simulink library "mesh_assembly_library"  (R2021a)
settings: Solver=VariableStepAuto  StartTime=0.0  StopTime=10.0  RelTol=1e-3
undefined symbols (not defined in the file): X, Y, Z
libraries: sm_lib x71, $bdroot x8, nesl_utility x6, Contact_Forces_Lib x1
(part 1 of 3)
settings Model: Creator=Daniel Adejumo  LastModifiedBy=Daniel Adejumo

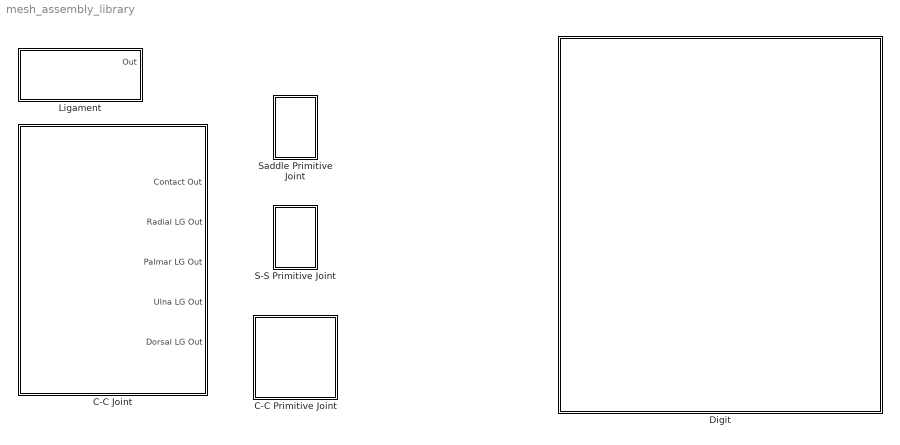
== system mesh_assembly_library ==
  C-C Joint : Subsystem  mask(Cylinder in Cylinder - DARM IP Joint){distal_arc_radius=0, proximal_arc_radius=0, active_range=[-60, 60], initial_rotation=0, distal_ring_thickness=1/1000, distal_surface_length=10/1000, distal_surface_thickness=0.1/1000, proximal_surface_length=10/1000, proximal_surface_thickness=0.1/1000, visual_color=[0.9 0.2 0.2], visual_opacity=0.7, contact_stiffness=1e4, contact_damping=1e2, coefficient_kinetic_friction=0.1, coefficient_static_friction=0.2, velocity_threshold=0.001, lg_tension_stiffness=0, lg_tension_damping_coefficient=0, lg_transition_region_width=1e-3, lg_density=0, lg_damping=0, radial_lg_dim=[0, 0, 0], palmar_lg_dim=[0, 0, 0], ulnar_lg_dim=[0, 0, 0], dorsal_lg_dim=[0, 0, 0]}
      mask prompts: distal_arc_radius "Distal Arc Radius [m]"; proximal_arc_radius "Proximal Arc Radius [m]"; active_range "Active Range (min, max angle) [deg]"; initial_rotation "Initial Rotation [deg]"; distal_ring_thickness "Distal Ring Thickness [m]"; distal_surface_length "Distal Surface Length [m]"; distal_surface_thickness "Distal Surface Thickness [m]"; proximal_surface_length "Proximal Surface Length [m]"; proximal_surface_thickness "Proximal Surface Thickness [m]"; visual_color "Visual Colour [RGB]"; visual_opacity "Visual Opacity (0 - 1)"; contact_stiffness "Contact Stiffness [N/m]"; contact_damping "Contact Damping [N/(m/s)]"; coefficient_kinetic_friction "Coefficient of Kinetic Friction"; coefficient_static_friction "Coefficient of Static Friction"; velocity_threshold "Velocity Threshold [m/s]"; lg_tension_stiffness "Tension Stiffness [N/m]"; lg_tension_damping_coefficient "Tension Damping Coefficient [N/(m/s)]"; lg_transition_region_width "Transition Region Width [m]"; lg_density "Density [Kg/m^3]"; lg_damping "Damping [N/(m/s)]"; radial_lg_dim "Dimensions (L, W, T) [m]"; palmar_lg_dim "Dimensions (L, W, T) [m]"; ulnar_lg_dim "Dimensions (L, W, T) [m]"; dorsal_lg_dim "Dimensions (L, W, T) [m]"
      mask help: The Cylinder in Cylinder Joint models a 1-DOF joint found in the interphalangeal articulation.
      settings: PortSchema="{\"entries\":[{\"content\":{\"sides\":[{\"content\":{\"connectorIds\":[\"LConn1\",\"LConn2\",\"LConn3\",\"LConn4\",\"LConn5\",\"LConn6\",\"LConn7\",\"LConn8\"]},\"type\":\"ConnectorPlacement.EquallySpacedRectSide\",\"uuid\":\"de75d0fa-dcb7-4671-a193-b6d8e2533622\"},{\"content\":{\"connectorIds\":[\"RConn1\",\"Out1\",\"Out2\",\"Out3\",\"Out4\",\"Out5\",\"RConn2\"],\"side\":\"RIGHT\"},\"type\":\"ConnectorPlacement.EquallySpacedRectSide\",\"uuid\":\"61947ab9-5bc1-4fe7-b694-bbba1acc34a0\"},{\"content\":{\"connectorIds\":[],\"side\":\"TOP\"},\"type\":\"ConnectorPlacement.EquallySpacedRectSide\",\"uuid\":\"94257d25-1dd3-43a0-827d-d6eeaffa38d1\"}]},\"type\":\"ConnectorPlacement.EquallySpacedConnector\",\"uuid\":\"ad636cf9-9422-4be4-a938-719e0f4b0058\"}],\"packageUris\":[\"http://schema.mathworks.com/mf0/Connector/R2020b\"],\"version\":\"1.0\"}"
      mask Help:
      | <p>The Cylinder in Cylinder Joint models a 1-DOF joint found in the interphalangeal articulation. </p>
      | 
      | <h3> Port Names: </h3>
      | 
      | <p><i>Radial LG Head_R:</i> Radial aspect of the head of the radial ligament</p>
      | <p><i>Radial LG Head_U:</i> Ulnar aspect of the head of the radial ligament</p>
      mask DialogControl DescGroupVar Prompt: Cylinder in Cyclinder Joint
      mask DialogControl DescTextVar Prompt: The Distal Arc Radius is the radius of its inner circle. The Proximal arc radius is the radius of its outer circle.
      mask DialogControl geometry Prompt: Geometry
      mask DialogControl visual Prompt: Visual
      mask DialogControl contact Prompt: Contact
      mask DialogControl Container13 Prompt: Ligaments
      mask DialogControl Container21 Prompt: Mechanics
      mask DialogControl Container20 Prompt: Geometry
      mask DialogControl Container16 Prompt: Radial Collateral Ligament
      mask DialogControl Container16_copy Prompt: Palmar Ligament
      mask DialogControl Container16_copy_copy Prompt: Ulnar Collateral Ligament
      mask DialogControl Container16_copy_copy_copy Prompt: Dorsal Ligament
  C-C Primitive Joint : Subsystem  mask{stiffness=0, damping=0, lower_limit=-90, upper_limit=90, initial_position=0, radius=0, length=0, thickness=0, color=[1.0 0.0 0.0], opacity=1.0}
      mask prompts: stiffness "Stiffness [Nm/deg]"; damping "Damping [Nm/(deg/s)]"; lower_limit "Lower Limit [deg]"; upper_limit "Upper Limit [deg]"; initial_position "Initial Position [deg]"; radius "Radius [m]"; length "Length [m]"; thickness "Thickness [m]"; color "Color (RGB - Range [0, 1])"; opacity "Opacity (Range [0, 1])"
      mask DialogControl DescGroupVar Prompt: C-C Primitive Joint
      mask DialogControl DescTextVar Prompt: Primitive representation of a cylinder to cylinder joint using a simple revolute joint. This joint is found in at the PIP and DIP joints.
      mask DialogControl Container4 Prompt: Mechanics
      mask DialogControl Container6 Prompt: Visualization
  Digit : Subsystem  mask{links_density=1000, distal_phalanx="", distal_phalanx_base=[[0 0 0]; [0 0 0]], distal_phalanx_dip_joint=[[0 0 0]; [0 0 0]], distal_phalanx_head=[[0 0 0]; [0 0 0]], middle_phalanx="", middle_phalanx_base=[[0 0 0]; [0 0 0]], middle_phalanx_pip_joint=[[0 0 0]; [0 0 0]], middle_phalanx_head=[[0 0 0]; [0 0 0]], middle_phalanx_dip_joint=[[0 0 0]; [0 0 0]], proximal_phalanx="", proximal_phalanx_base=[[0 0 0]; [0 0 0]], proximal_phalanx_mcp_joint=[[0 0 0]; [0 0 0]], proximal_phalanx_head=[[0 0 0]; [0 0 0]], proximal_phalanx_pip_joint=[[0 0 0]; [0 0 0]], metacarpal="", metacarpal_base=[[0 0 0]; [0 0 0]], metacarpal_cm_joint=[[0 0 0]; [0 0 0]], metacarpal_head=[[0 0 0]; [0 0 0]], metacarpal_mcp_joint=[[0 0 0]; [0 0 0]], mcp_viz_radius=0, mcp_viz_color=[1.0 0.0 0.0], mcp_viz_opacity=1.0, pip_viz_radius=0, pip_viz_length=0, pip_viz_thickness=0, pip_viz_color=[1.0 0.0 0.0], pip_viz_opacity=1.0, dip_viz_radius=0, dip_viz_length=0, dip_viz_thickness=0, dip_viz_color=[1.0 0.0 0.0], dip_viz_opacity=1.0}
      mask prompts: links_density "Density [Kg/(m^3)]"; distal_phalanx "File Name"; distal_phalanx_base "Base Transform (Translation [m], Rotation: X-Y-Z [deg])"; distal_phalanx_dip_joint "DIP Joint Transform (Translation, Rotation)"; distal_phalanx_head "Head Transform (Translation, Rotation)"; middle_phalanx "File Name"; middle_phalanx_base "Base Transform"; middle_phalanx_pip_joint "PIP Joint Transform"; middle_phalanx_head "Head Transform"; middle_phalanx_dip_joint "DIP Joint Transform"; proximal_phalanx "File Name"; proximal_phalanx_base "Base Transform"; proximal_phalanx_mcp_joint "MCP Joint Transform"; proximal_phalanx_head "Head Transform"; proximal_phalanx_pip_joint "PIP Joint Transform"; metacarpal "File Name"; metacarpal_base "Base Transform"; metacarpal_cm_joint "CM Joint Transform"; metacarpal_head "Head Transform"; metacarpal_mcp_joint "MCP Joint Transform"; mcp_viz_radius "Radius [m]"; mcp_viz_color "Color (RGB - Range [0, 1])"; mcp_viz_opacity "Opacity (Range [0, 1])"; pip_viz_radius "Radius [m]"; pip_viz_length "Length [m]"; pip_viz_thickness "Thickness [m]"; pip_viz_color "Color (RGB - Range [0, 1])"; pip_viz_opacity "Opacity (Range [0, 1])"; dip_viz_radius "Radius [m]"; dip_viz_length "Length [m]"; dip_viz_thickness "Thickness [m]"; dip_viz_color "Color (RGB - Range [0, 1])"; dip_viz_opacity "Opacity (Range [0, 1])"
      mask DialogControl DescGroupVar Prompt: Digit Subsystem
      mask DialogControl DescTextVar Prompt: This subsystem encapsulates the bones and joints that makes up digits II - V. Metacarpal bone, Proximal, Middle and Distal Phalanxes; MCP, PIP and DIP Joints.
      mask DialogControl Links Prompt: Links
      mask DialogControl Distal_Phalanx Prompt: Distal Phalanx
      mask DialogControl Middle_Phalanx Prompt: Middle Phalanx
      mask DialogControl Proximal_Phalanx Prompt: Proximal Phalanx
      mask DialogControl Metacarpal Prompt: Metacarpal
      mask DialogControl Container10 Prompt: Visualization
      mask DialogControl Container11 Prompt: MCP Joint
      mask DialogControl Container12 Prompt: PIP Joint
      mask DialogControl Container13 Prompt: DIP Joint
  Ligament : Subsystem  Variant=on  mask{length=0.4, width=0.08, thickness=0.008, tension_stiffness=35E3, tension_damping_coefficient=100, transition_region_width=1e-3, density=800, damping_coefficient=0.2}
      mask prompts: length "Length [m]"; width "Width [m]"; thickness "Thickness [m]"; tension_stiffness "Tension Stiffness [N/m]"; tension_damping_coefficient "Tension Damping Coefficient [N/(m/s)]"; transition_region_width "Transition Region Width [m]"; density "Density [Kg/m^3]"; damping_coefficient "Damping [N/(m/s)]"
      mask DialogControl geometry Prompt: Geometry Parameters
      mask DialogControl mechanics Prompt: Mechanics Parameters
  S-S Primitive Joint : Subsystem  mask{stiffness=0, damping=0, x_limits=[-90 90], y_limits=[-90 90], x_initial_position=0, y_initial_position=0, radius=0, color=[1.0 0.0 0.0], opacity=1.0}
      mask prompts: x_limits "X Limits"; y_limits "Y Limits"; x_initial_position "X Initial Position"; y_initial_position "Y Initial Position"; radius "Radius [m]"; color "Color (RGB - Range [0, 1])"; opacity "Opacity (Range [0, 1])"
      mask DialogControl DescGroupVar Prompt: S-S Primitive Joint
      mask DialogControl DescTextVar Prompt: Primitive representation of the sphere to sphere joint using a universal joint. This is found at the MCP joints.
      mask DialogControl Container4 Prompt: Mechanics
      mask DialogControl Container6 Prompt: Visualization
  Saddle Primitive Joint : Subsystem  mask{stiffness=0, damping=0, x_limits=[-90 90], y_limits=[-90 90], z_limits=[-90 90], x_initial_position=0, y_initial_position=0, z_initial_position=0, centre_block_dim=[1, 1, 12]/1000, centre_block_density=0, thickness=0.5/1000, x_radius=0, x_length=0, x_color=[1.0 0.0 0.0], x_opacity=1.0, y_radius=0, y_length=0, y_color=[1.0 0.0 0.0], y_opacity=1.0, z_radius=0, z_length=0, z_color=[1.0 0.0 0.0], z_opacity=1.0}
      mask prompts: stiffness "Stiffness [N*m/deg]"; damping "Damping [N*m/(deg/s)]"; x_limits "X Limits (low, high) [deg]"; y_limits "Y Limits (low, high) [deg]"; z_limits "Z Limits (low, high) [deg]"; x_initial_position "X Initial Position [deg]"; y_initial_position "Y Initial Position [deg]"; z_initial_position "Z Initial Position [deg]"; centre_block_dim "Centre Block Dimension [m]"; centre_block_density "Ignore this Param"; thickness "Thickness [m]"; x_radius "X Radius [m]"; x_length "X Length [m]"; x_color "X Color (RGB - Range [0, 1])"; x_opacity "X Opacity (Range [0, 1])"; y_radius "Y Radius [m]"; y_length "Y Length [m]"; y_color "Y Color (RGB - Range [0, 1])"; y_opacity "X Opacity (Range [0, 1])"; z_radius "Z Radius [m]"; z_length "Z Length [m]"; z_color "Z Color (RGB - Range [0, 1])"; z_opacity "Z Opacity (Range [0, 1])"
      mask DialogControl DescGroupVar Prompt: Saddle Primitive Joint
      mask DialogControl DescTextVar Prompt: Primitive representation of the Saddle Joint using a Gimbal Joint. This is found at the MCP joint of the thumb.
      mask DialogControl Container10 Prompt: Mechanics
      mask DialogControl Container4 Prompt: Visualization
      mask DialogControl Container6 Prompt: X Axis
      mask DialogControl Container7 Prompt: Y Axis
      mask DialogControl Container8 Prompt: Z Axis

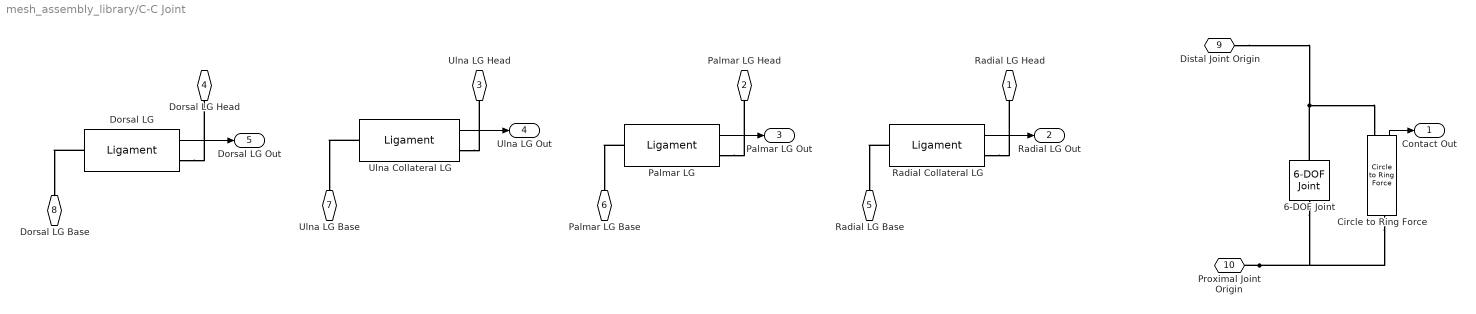
== system mesh_assembly_library/C-C Joint ==
  6-DOF Joint : sm_lib/Joints/6-DOF Joint  JointMode=Normal  SenseConstraintForce=off  SenseConstraintForceX=off  SenseConstraintForceY=off  SenseConstraintForceZ=off  SenseConstraintTorque=off  SenseConstraintTorqueX=off  SenseConstraintTorqueY=off  SenseConstraintTorqueZ=off  SenseTotalForce=off  SenseTotalForceX=off  SenseTotalForceY=off  SenseTotalForceZ=off  SenseTotalTorque=off  SenseTotalTorqueX=off  SenseTotalTorqueY=off  SenseTotalTorqueZ=off  CompositeWrenchDir=FollowerOnBase  CompositeWrenchFrame=BaseFrame  PxEquilibriumPosition=0  PxEquilibriumPositionUnits=m  PxSpringStiffness=0  PxSpringStiffnessUnits=N/m  PxDampingCoefficient=0  PxDampingCoefficientUnits=N/(m/s)  PxTorqueActuationMode=NoTorque  PxMotionActuationMode=ComputedMotion  PxSensePosition=off  PxSenseVelocity=off  PxSenseAcceleration=off  PxSenseTorqueForce=off  PxSenseLowerLimitTorqueForce=off  PxSenseUpperLimitTorqueForce=off  PxLowerLimitSpecify=off  PxLowerLimitBound=-1  PxLowerLimitBoundUnits=m  PxLowerLimitStiffness=1e6  PxLowerLimitStiffnessUnits=N/m  PxLowerLimitDamping=1e3  PxLowerLimitDampingUnits=N/(m/s)  PxLowerLimitTransitionRegionWidth=1e-4  PxLowerLimitTransitionRegionWidthUnits=m  PxUpperLimitSpecify=off  PxUpperLimitBound=1  PxUpperLimitBoundUnits=m  PxUpperLimitStiffness=1e6  PxUpperLimitStiffnessUnits=N/m  PxUpperLimitDamping=1e3  PxUpperLimitDampingUnits=N/(m/s)  PxUpperLimitTransitionRegionWidth=1e-4  PxUpperLimitTransitionRegionWidthUnits=m  PxPositionTargetSpecify=on  PxPositionTargetPriority=High  PxPositionTargetValue=0  PxPositionTargetValueUnits=m  PxVelocityTargetSpecify=off  PxVelocityTargetPriority=High  PxVelocityTargetValue=0  PxVelocityTargetValueUnits=m/s  PyEquilibriumPosition=0  PyEquilibriumPositionUnits=m  PySpringStiffness=0  PySpringStiffnessUnits=N/m  PyDampingCoefficient=0  PyDampingCoefficientUnits=N/(m/s)  PyTorqueActuationMode=NoTorque  PyMotionActuationMode=ComputedMotion  PySensePosition=off  PySenseVelocity=off  PySenseAcceleration=off  PySenseTorqueForce=off  PySenseLowerLimitTorqueForce=off  PySenseUpperLimitTorqueForce=off  PyLowerLimitSpecify=off  PyLowerLimitBound=-1  PyLowerLimitBoundUnits=m  PyLowerLimitStiffness=1e6  PyLowerLimitStiffnessUnits=N/m  PyLowerLimitDamping=1e3  PyLowerLimitDampingUnits=N/(m/s)  PyLowerLimitTransitionRegionWidth=1e-4  PyLowerLimitTransitionRegionWidthUnits=m  PyUpperLimitSpecify=off  PyUpperLimitBound=1  PyUpperLimitBoundUnits=m  PyUpperLimitStiffness=1e6  PyUpperLimitStiffnessUnits=N/m  PyUpperLimitDamping=1e3  PyUpperLimitDampingUnits=N/(m/s)  PyUpperLimitTransitionRegionWidth=1e-4  PyUpperLimitTransitionRegionWidthUnits=m  PyPositionTargetSpecify=on  PyPositionTargetPriority=High  PyPositionTargetValue=0  PyPositionTargetValueUnits=m  PyVelocityTargetSpecify=off  PyVelocityTargetPriority=High  PyVelocityTargetValue=0  PyVelocityTargetValueUnits=m/s  PzEquilibriumPosition=0  PzEquilibriumPositionUnits=m  PzSpringStiffness=0  PzSpringStiffnessUnits=N/m  PzDampingCoefficient=0  PzDampingCoefficientUnits=N/(m/s)  PzTorqueActuationMode=NoTorque  PzMotionActuationMode=ComputedMotion  PzSensePosition=off  PzSenseVelocity=off  PzSenseAcceleration=off  PzSenseTorqueForce=off  PzSenseLowerLimitTorqueForce=off  PzSenseUpperLimitTorqueForce=off  PzLowerLimitSpecify=off  PzLowerLimitBound=-1  PzLowerLimitBoundUnits=m  PzLowerLimitStiffness=1e6  PzLowerLimitStiffnessUnits=N/m  PzLowerLimitDamping=1e3  PzLowerLimitDampingUnits=N/(m/s)  PzLowerLimitTransitionRegionWidth=1e-4  PzLowerLimitTransitionRegionWidthUnits=m  PzUpperLimitSpecify=off  PzUpperLimitBound=1  PzUpperLimitBoundUnits=m  PzUpperLimitStiffness=1e6  PzUpperLimitStiffnessUnits=N/m  PzUpperLimitDamping=1e3  PzUpperLimitDampingUnits=N/(m/s)  PzUpperLimitTransitionRegionWidth=1e-4  PzUpperLimitTransitionRegionWidthUnits=m  PzPositionTargetSpecify=on  PzPositionTargetPriority=High  PzPositionTargetValue=0  PzPositionTargetValueUnits=m  PzVelocityTargetSpecify=off  PzVelocityTargetPriority=High  PzVelocityTargetValue=0  PzVelocityTargetValueUnits=m/s  SphDefPosRotationMethod=None  SphDefPosRotationAngleUnits=deg  SphDefPosRotationStandardAxis=+Z  SphDefPosRotationAngle=0.0  SphDefPosRotationArbitraryAxis=[0 0 1]  SphDefPosFollAlignAxisA=+X  SphDefPosBaseAlignAxisA=+Y  SphDefPosFollAlignAxisB=+Y  SphDefPosBaseAlignAxisB=+Z  SphDefPosRotationSequenceAxes=FollowerAxes  SphDefPosRotationSequence=XYX  SphDefPosRotationSequenceAngles=[0 0 0]  SphDefPosRotationSequenceAnglesUnits=deg  SphDefPosRotationMatrix=[1 0 0; 0 1 0; 0 0 1]  SphEqPosRotationMethod=None  SphEqPosRotationAngleUnits=deg  SphEqPosRotationStandardAxis=+Z  SphEqPosRotationAngle=0.0  SphEqPosRotationArbitraryAxis=[0 0 1]  SphEqPosFollAlignAxisA=+X  SphEqPosBaseAlignAxisA=+Y  SphEqPosFollAlignAxisB=+Y  SphEqPosBaseAlignAxisB=+Z  SphEqPosRotationSequenceAxes=FollowerAxes  SphEqPosRotationSequence=XYX  SphEqPosRotationSequenceAngles=[0 0 0]  SphEqPosRotationSequenceAnglesUnits=deg  SphEqPosRotationMatrix=[1 0 0; 0 1 0; 0 0 1]  SphSpringStiffness=0  SphSpringStiffnessUnits=N*m/deg  SphDampingCoefficient=0  SphDampingCoefficientUnits=N*m/(deg/s)  SphActuateTorqueX=off  SphActuateTorqueY=off  SphActuateTorqueZ=off  SphActuateTorque=off  SphTorqueActuationMode=NoTorque  SphMotionActuationMode=ComputedMotion  SphActuationFrame=BaseFrame  SphSensePosition=off  SphSenseVelocityX=off  SphSenseVelocityY=off  SphSenseVelocityZ=off  SphSenseVelocity=off  SphSenseAccelerationX=off  SphSenseAccelerationY=off  SphSenseAccelerationZ=off  SphSenseAcceleration=off  SphSenseTorqueX=off  SphSenseTorqueY=off  SphSenseTorqueZ=off  SphSenseTorqueForce=off  SphSenseLowerLimitTorqueMag=off  SphSenseUpperLimitTorqueMag=off  SphSensingFrame=BaseFrame  SphLowerLimitSpecify=off  SphLowerLimitBound=15  SphLowerLimitBoundUnits=deg  SphLowerLimitStiffness=1e4  SphLowerLimitStiffnessUnits=N*m/deg  SphLowerLimitDamping=10  SphLowerLimitDampingUnits=N*m/(deg/s)  SphLowerLimitTransitionRegionWidth=0.1  SphLowerLimitTransitionRegionWidthUnits=deg  SphUpperLimitSpecify=off  SphUpperLimitBound=45  SphUpperLimitBoundUnits=deg  SphUpperLimitStiffness=1e4  SphUpperLimitStiffnessUnits=N*m/deg  SphUpperLimitDamping=10  SphUpperLimitDampingUnits=N*m/(deg/s)  SphUpperLimitTransitionRegionWidth=0.1  SphUpperLimitTransitionRegionWidthUnits=deg  SphPositionTargetRotationMethod=RotationSequence  SphPositionTargetRotationAngleUnits=deg  SphPositionTargetRotationStandardAxis=+Z  SphPositionTargetRotationAngle=0.0  SphPositionTargetRotationArbitraryAxis=[0 0 1]  SphPositionTargetFollAlignAxisA=+X  SphPositionTargetBaseAlignAxisA=+X  SphPositionTargetFollAlignAxisB=+Y  SphPositionTargetBaseAlignAxisB=+Y  SphPositionTargetRotationSequenceAxes=FollowerAxes  SphPositionTargetRotationSequence=XYZ  SphPositionTargetRotationSequenceAngles=[0 0 initial_rotation]  SphPositionTargetRotationSequenceAnglesUnits=deg  SphPositionTargetRotationMatrix=[1 0 0; 0 1 0; 0 0 1]  SphPositionTargetSpecify=on  SphPositionTargetPriority=High  SphVelocityTargetValue=[0 0 0]  SphVelocityTargetValueUnits=deg/s  SphVelocityTargetSpecify=off  SphVelocityTargetPriority=High  SphVelocityTargetInFollowerFrame=on
  Circle to Ring Force : Contact_Forces_Lib/2D/Circle to Ring Force  radius_circle=proximal_arc_radius  radius_ring=distal_arc_radius + (distal_ring_thickness/2)  d_ring=distal_ring_thickness  active_angle=active_range  force_law=Linear  k_contact=contact_stiffness  b_contact=contact_damping  pen_full_damp_F=1e-4  pen_exponent=1  custom_param_1=1  custom_param_2=1  friction_law=Stick-Slip Continuous  mu_kinetic=coefficient_kinetic_friction  mu_static=coefficient_static_friction  v_thr=velocity_threshold  vis_on=on  vis_opc_en=0  vis_len_rinBz=distal_surface_length  vis_len_rinBx=distal_surface_thickness  vis_len_cirFz=proximal_surface_length  vis_len_cirFx=proximal_surface_thickness  vis_clr=visual_color  vis_opc=visual_opacity
  Dorsal LG : $bdroot/Ligament  length=dorsal_lg_dim(1)  width=dorsal_lg_dim(2)  thickness=dorsal_lg_dim(3)  tension_stiffness=lg_tension_stiffness  tension_damping_coefficient=lg_tension_damping  transition_region_width=lg_transition_region_width  density=lg_density  damping_coefficient=lg_damping
  Palmar LG : $bdroot/Ligament  length=palmar_lg_dim(1)  width=palmar_lg_dim(2)  thickness=palmar_lg_dim(3)  tension_stiffness=lg_tension_stiffness  tension_damping_coefficient=lg_tension_damping  transition_region_width=lg_transition_region_width  density=lg_density  damping_coefficient=lg_damping
  Radial Collateral LG : $bdroot/Ligament  length=radial_lg_dim(1)  width=radial_lg_dim(2)  thickness=radial_lg_dim(3)  tension_stiffness=lg_tension_stiffness  tension_damping_coefficient=lg_tension_damping  transition_region_width=lg_transition_region_width  density=lg_density  damping_coefficient=lg_damping
  Ulna Collateral LG : $bdroot/Ligament  length=ulnar_lg_dim(1)  width=ulnar_lg_dim(2)  thickness=ulnar_lg_dim(3)  tension_stiffness=lg_tension_stiffness  tension_damping_coefficient=lg_tension_damping  transition_region_width=lg_transition_region_width  density=lg_density  damping_coefficient=lg_damping
  Radial LG Head : PMIOPort  Side=Left
  Palmar LG Head : PMIOPort  Port=2  Side=Left
  Ulna LG Head : PMIOPort  Port=3  Side=Left
  Dorsal LG Head : PMIOPort  Port=4  Side=Left
  Radial LG Base : PMIOPort  Port=5  Side=Left
  Palmar LG Base : PMIOPort  Port=6  Side=Left
  Ulna LG Base : PMIOPort  Port=7  Side=Left
  Dorsal LG Base : PMIOPort  Port=8  Side=Left
  Distal Joint Origin : PMIOPort  Port=9  Side=Right
  Proximal Joint Origin : PMIOPort  Port=10  Side=Right
  Contact Out : Outport
  Radial LG Out : Outport  Port=2
  Palmar LG Out : Outport  Port=3
  Ulna LG Out : Outport  Port=4
  Dorsal LG Out : Outport  Port=5
  wires:
  Circle to Ring Force/1 -> Contact Out/1
  Palmar LG/1 -> Palmar LG Out/1
  Radial Collateral LG/1 -> Radial LG Out/1
  Ulna Collateral LG/1 -> Ulna LG Out/1
  Dorsal LG/1 -> Dorsal LG Out/1
  connections:
  Ulna Collateral LG/RConn1 -- Ulna LG Head/RConn1
  Palmar LG/RConn1 -- Palmar LG Head/RConn1
  Dorsal LG/LConn1 -- Dorsal LG Base/RConn1
  Radial Collateral LG/LConn1 -- Radial LG Base/RConn1
  Ulna Collateral LG/LConn1 -- Ulna LG Base/RConn1
  Radial Collateral LG/RConn1 -- Radial LG Head/RConn1
  Proximal Joint Origin/RConn1 -- Circle to Ring Force/LConn1 -- 6-DOF Joint/LConn1
  Palmar LG/LConn1 -- Palmar LG Base/RConn1
  Distal Joint Origin/RConn1 -- Circle to Ring Force/RConn1 -- 6-DOF Joint/RConn1
  Dorsal LG/RConn1 -- Dorsal LG Head/RConn1

== system mesh_assembly_library/C-C Primitive Joint ==
  Revolute Joint : sm_lib/Joints/Revolute Joint  JointMode=Normal  SenseConstraintForce=off  SenseConstraintForceX=off  SenseConstraintForceY=off  SenseConstraintForceZ=off  SenseConstraintTorque=off  SenseConstraintTorqueX=off  SenseConstraintTorqueY=off  SenseConstraintTorqueZ=off  SenseTotalForce=off  SenseTotalForceX=off  SenseTotalForceY=off  SenseTotalForceZ=off  SenseTotalTorque=off  SenseTotalTorqueX=off  SenseTotalTorqueY=off  SenseTotalTorqueZ=off  CompositeWrenchDir=FollowerOnBase  CompositeWrenchFrame=BaseFrame  EquilibriumPosition=0  EquilibriumPositionUnits=deg  SpringStiffness=stiffness  SpringStiffnessUnits=N*m/deg  DampingCoefficient=damping  DampingCoefficientUnits=N*m/(deg/s)  TorqueActuationMode=NoTorque  MotionActuationMode=ComputedMotion  SensePosition=off  SenseVelocity=off  SenseAcceleration=off  SenseTorqueForce=off  SenseLowerLimitTorqueForce=off  SenseUpperLimitTorqueForce=off  LowerLimitSpecify=on  LowerLimitBound=lower_limit  LowerLimitBoundUnits=deg  LowerLimitStiffness=1e4  LowerLimitStiffnessUnits=N*m/deg  LowerLimitDamping=10  LowerLimitDampingUnits=N*m/(deg/s)  LowerLimitTransitionRegionWidth=0.1  LowerLimitTransitionRegionWidthUnits=deg  UpperLimitSpecify=on  UpperLimitBound=upper_limit  UpperLimitBoundUnits=deg  UpperLimitStiffness=1e4  UpperLimitStiffnessUnits=N*m/deg  UpperLimitDamping=10  UpperLimitDampingUnits=N*m/(deg/s)  UpperLimitTransitionRegionWidth=0.1  UpperLimitTransitionRegionWidthUnits=deg  PositionTargetSpecify=on  PositionTargetPriority=High  PositionTargetValue=initial_position  PositionTargetValueUnits=deg  VelocityTargetSpecify=off  VelocityTargetPriority=High  VelocityTargetValue=0  VelocityTargetValueUnits=deg/s
  X Axis_B Transform : sm_lib/Frames and Transforms/Rigid Transform  TranslationMethod=None  TranslationStandardOffset=0  TranslationLengthUnit=m  TranslationStandardAxis=+Z  TranslationCartesianOffset=[0 0 0]  TranslationROffset=0  TranslationROffsetUnits=m  TranslationZOffset=0  TranslationZOffsetUnits=m  TranslationThetaOffset=0  TranslationThetaOffsetUnits=deg  RotationMethod=AlignedAxes  RotationAngleUnits=deg  RotationStandardAxis=+Z  RotationAngle=0.0  RotationArbitraryAxis=[0 0 1]  FollAlignAxisA=+Z  BaseAlignAxisA=+X  FollAlignAxisB=+X  BaseAlignAxisB=+Z  RotationSequenceAxes=FollowerAxes  RotationSequence=XYX  RotationSequenceAngles=[0 0 0]  RotationSequenceAnglesUnits=deg  RotationMatrix=[1 0 0; 0 1 0; 0 0 1]
  X Axis_F Transform1 : sm_lib/Frames and Transforms/Rigid Transform  TranslationMethod=None  TranslationStandardOffset=0  TranslationLengthUnit=m  TranslationStandardAxis=+Z  TranslationCartesianOffset=[0 0 0]  TranslationROffset=0  TranslationROffsetUnits=m  TranslationZOffset=0  TranslationZOffsetUnits=m  TranslationThetaOffset=0  TranslationThetaOffsetUnits=deg  RotationMethod=AlignedAxes  RotationAngleUnits=deg  RotationStandardAxis=+Z  RotationAngle=0.0  RotationArbitraryAxis=[0 0 1]  FollAlignAxisA=+Z  BaseAlignAxisA=+X  FollAlignAxisB=+X  BaseAlignAxisB=+Z  RotationSequenceAxes=FollowerAxes  RotationSequence=XYX  RotationSequenceAngles=[0 0 0]  RotationSequenceAnglesUnits=deg  RotationMatrix=[1 0 0; 0 1 0; 0 0 1]
  X_Viz axis Transform : sm_lib/Frames and Transforms/Rigid Transform  TranslationMethod=None  TranslationStandardOffset=0  TranslationLengthUnit=m  TranslationStandardAxis=+Z  TranslationCartesianOffset=[0 0 0]  TranslationROffset=0  TranslationROffsetUnits=m  TranslationZOffset=0  TranslationZOffsetUnits=m  TranslationThetaOffset=0  TranslationThetaOffsetUnits=deg  RotationMethod=AlignedAxes  RotationAngleUnits=deg  RotationStandardAxis=+Z  RotationAngle=0.0  RotationArbitraryAxis=[0 0 1]  FollAlignAxisA=+Z  BaseAlignAxisA=+X  FollAlignAxisB=+X  BaseAlignAxisB=+Z  RotationSequenceAxes=FollowerAxes  RotationSequence=XYX  RotationSequenceAngles=[0 0 0]  RotationSequenceAnglesUnits=deg  RotationMatrix=[1 0 0; 0 1 0; 0 0 1]
  X_Viz_Cylinder : sm_lib/Body Elements/Revolved Solid  GraphicAmbientColor=[0.15 0.15 0.15 1.0]  BasedOnType=Mass  CenterOfMass=[0 0 0]  CenterOfMassUnits=m  GraphicDiffuseColor=color  ExportConvexHullGeometry=off  Density=1000  DensityUnits=kg/m^3  DoExposeReferenceFrame=on  GraphicEmissiveColor=[0.0 0.0 0.0 1.0]  ExportEntireGeometry=off  SerializedFrames=<Frames/>  MarkerShape=Sphere  MarkerSize=10  GraphicType=FromGeometry  InertiaType=CalculateFromGeometry  Mass=0  MassUnits=kg  MomentsOfInertia=[1 1 1]  MomentsOfInertiaUnits=kg*m^2  GraphicOpacity=opacity  ProductsOfInertia=[0 0 0]  ProductsOfInertiaUnits=kg*m^2  RevolutionCrossSection=|  RevolutionCrossSectionUnits=m  RevolutionAngle=180  RevolutionAngleUnits=deg  RevolutionExtent=Full  GraphicShininess=75  GraphicSpecularColor=[0.5 0.5 0.5 1.0]  GraphicVisPropType=SimpleVisualProperties
      | [radius, length/2;
      |  radius, -length/2;
      |  radius+thickness, -length/2;
      |  radius+thickness, length/2]
  F : PMIOPort  Side=Right
  B : PMIOPort  Port=2  Side=Left
  connections:
  X Axis_F Transform1/LConn1 -- F/RConn1
  X Axis_F Transform1/RConn1 -- Revolute Joint/RConn1
  Revolute Joint/LConn1 -- X Axis_B Transform/RConn1
  X Axis_B Transform/LConn1 -- B/RConn1 -- X_Viz axis Transform/LConn1
  X_Viz_Cylinder/RConn1 -- X_Viz axis Transform/RConn1

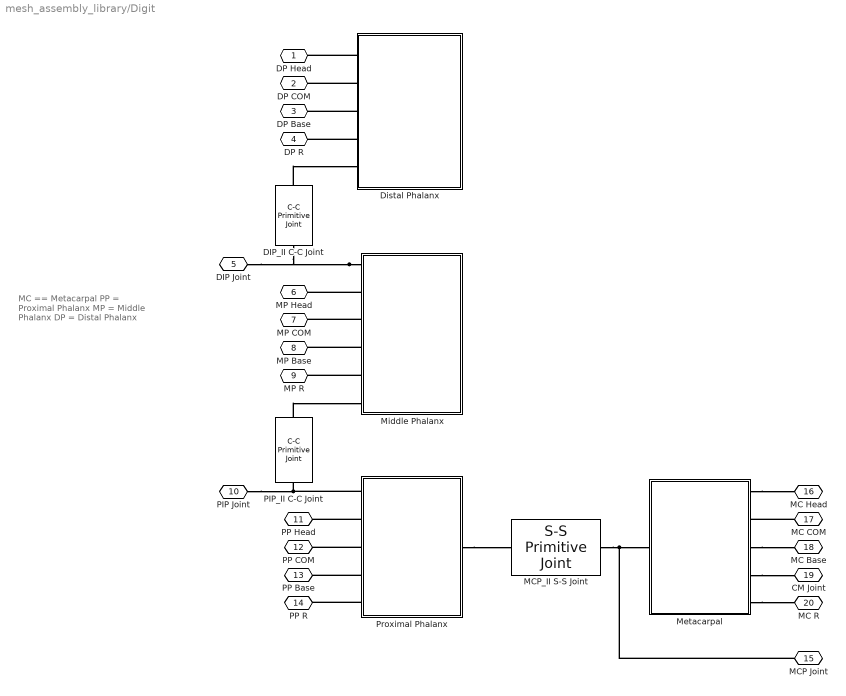
== system mesh_assembly_library/Digit ==
  note: MC == Metacarpal
      | PP = Proximal Phalanx
      | MP = Middle Phalanx
      | DP = Distal Phalanx
  DIP_II C-C Joint : $bdroot/C-C Primitive Joint  stiffness=0  damping=0  lower_limit=-90  upper_limit=90  initial_position=0  radius=dip_viz_radius  length=dip_viz_length  thickness=dip_viz_thickness  color=dip_viz_color  opacity=dip_viz_opacity
  Distal Phalanx : Subsystem
  MCP_II S-S Joint : $bdroot/S-S Primitive Joint  stiffness=0  damping=0  x_limits=[-90 90]  y_limits=[-90 90]  x_initial_position=0  y_initial_position=0  radius=mcp_viz_radius  color=mcp_viz_color  opacity=mcp_viz_opacity
  Metacarpal : Subsystem
  Middle Phalanx : Subsystem
  PIP_II C-C Joint : $bdroot/C-C Primitive Joint  stiffness=0  damping=0  lower_limit=-90  upper_limit=90  initial_position=0  radius=pip_viz_radius  length=pip_viz_length  thickness=pip_viz_thickness  color=pip_viz_color  opacity=pip_viz_opacity
  Proximal Phalanx : Subsystem
  DP Head : PMIOPort  Side=Left
  DP COM : PMIOPort  Port=2  Side=Left
  DP Base : PMIOPort  Port=3  Side=Left
  DP R : PMIOPort  Port=4  Side=Left
  DIP Joint : PMIOPort  Port=5  Side=Left
  MP Head : PMIOPort  Port=6  Side=Left
  MP COM : PMIOPort  Port=7  Side=Left
  MP Base : PMIOPort  Port=8  Side=Left
  MP R : PMIOPort  Port=9  Side=Left
  PIP Joint : PMIOPort  Port=10  Side=Left
  PP Head : PMIOPort  Port=11  Side=Left
  PP COM : PMIOPort  Port=12  Side=Left
  PP Base : PMIOPort  Port=13  Side=Left
  PP R : PMIOPort  Port=14  Side=Left
  MCP Joint : PMIOPort  Port=15  Side=Left
  MC Head : PMIOPort  Port=16  Side=Left
  MC COM : PMIOPort  Port=17  Side=Left
  MC Base : PMIOPort  Port=18  Side=Left
  CM Joint : PMIOPort  Port=19  Side=Left
  MC R : PMIOPort  Port=20  Side=Left
  connections:
  Proximal Phalanx/LConn5 -- PP R/RConn1
  Proximal Phalanx/LConn4 -- PP Base/RConn1
  Proximal Phalanx/LConn2 -- PP Head/RConn1
  Distal Phalanx/LConn1 -- DP Head/RConn1
  Distal Phalanx/LConn2 -- DP COM/RConn1
  Metacarpal/RConn5 -- MC R/RConn1
  Metacarpal/RConn1 -- MC Head/RConn1
  Metacarpal/RConn4 -- CM Joint/RConn1
  Metacarpal/RConn3 -- MC Base/RConn1
  Middle Phalanx/LConn4 -- MP Base/RConn1
  Middle Phalanx/LConn2 -- MP Head/RConn1
  PIP_II C-C Joint/RConn1 -- Middle Phalanx/LConn6
  Distal Phalanx/LConn4 -- DP R/RConn1
  MCP Joint/RConn1 -- MCP_II S-S Joint/LConn1 -- Metacarpal/LConn1
  Middle Phalanx/LConn3 -- MP COM/RConn1
  Proximal Phalanx/LConn3 -- PP COM/RConn1
  Middle Phalanx/LConn1 -- DIP_II C-C Joint/LConn1 -- DIP Joint/RConn1
  Middle Phalanx/LConn5 -- MP R/RConn1
  Distal Phalanx/LConn3 -- DP Base/RConn1
  Proximal Phalanx/RConn1 -- MCP_II S-S Joint/RConn1
  PIP Joint/RConn1 -- Proximal Phalanx/LConn1 -- PIP_II C-C Joint/LConn1
  DIP_II C-C Joint/RConn1 -- Distal Phalanx/LConn5
  MC COM/RConn1 -- Metacarpal/RConn2

== system mesh_assembly_library/Ligament ==
  note: 1) Add Subsystem or Model blocks as valid variant choices.
      | 2) You cannot connect blocks at this level. At simulation, connectivity is automatically
      | determined, based on the active variant and port name matching.
  Belt Cable : Subsystem  VariantControl=false
  Flexible Bodies : Subsystem  VariantControl=false
  Telescoping Joint : Subsystem  VariantControl=true
  Base : PMIOPort  Side=Left
  Head : PMIOPort  Port=2  Side=Right
  Out : Outport

== system mesh_assembly_library/S-S Primitive Joint ==
  Universal Joint : sm_lib/Joints/Universal Joint  JointMode=Normal  SenseConstraintForce=off  SenseConstraintForceX=off  SenseConstraintForceY=off  SenseConstraintForceZ=off  SenseConstraintTorque=off  SenseConstraintTorqueX=off  SenseConstraintTorqueY=off  SenseConstraintTorqueZ=off  SenseTotalForce=off  SenseTotalForceX=off  SenseTotalForceY=off  SenseTotalForceZ=off  SenseTotalTorque=off  SenseTotalTorqueX=off  SenseTotalTorqueY=off  SenseTotalTorqueZ=off  CompositeWrenchDir=FollowerOnBase  CompositeWrenchFrame=BaseFrame  RxEquilibriumPosition=0  RxEquilibriumPositionUnits=deg  RxSpringStiffness=stiffness  RxSpringStiffnessUnits=N*m/deg  RxDampingCoefficient=damping  RxDampingCoefficientUnits=N*m/(deg/s)  RxTorqueActuationMode=NoTorque  RxMotionActuationMode=ComputedMotion  RxSensePosition=off  RxSenseVelocity=off  RxSenseAcceleration=off  RxSenseTorqueForce=off  RxSenseLowerLimitTorqueForce=off  RxSenseUpperLimitTorqueForce=off  RxLowerLimitSpecify=on  RxLowerLimitBound=x_limits(1)  RxLowerLimitBoundUnits=deg  RxLowerLimitStiffness=1e4  RxLowerLimitStiffnessUnits=N*m/deg  RxLowerLimitDamping=10  RxLowerLimitDampingUnits=N*m/(deg/s)  RxLowerLimitTransitionRegionWidth=0.1  RxLowerLimitTransitionRegionWidthUnits=deg  RxUpperLimitSpecify=on  RxUpperLimitBound=x_limits(2)  RxUpperLimitBoundUnits=deg  RxUpperLimitStiffness=1e4  RxUpperLimitStiffnessUnits=N*m/deg  RxUpperLimitDamping=10  RxUpperLimitDampingUnits=N*m/(deg/s)  RxUpperLimitTransitionRegionWidth=0.1  RxUpperLimitTransitionRegionWidthUnits=deg  RxPositionTargetSpecify=on  RxPositionTargetPriority=High  RxPositionTargetValue=x_initial_position  RxPositionTargetValueUnits=deg  RxVelocityTargetSpecify=off  RxVelocityTargetPriority=High  RxVelocityTargetValue=0  RxVelocityTargetValueUnits=deg/s  RyEquilibriumPosition=0  RyEquilibriumPositionUnits=deg  RySpringStiffness=stiffness  RySpringStiffnessUnits=N*m/deg  RyDampingCoefficient=damping  RyDampingCoefficientUnits=N*m/(deg/s)  RyTorqueActuationMode=NoTorque  RyMotionActuationMode=ComputedMotion  RySensePosition=off  RySenseVelocity=off  RySenseAcceleration=off  RySenseTorqueForce=off  RySenseLowerLimitTorqueForce=off  RySenseUpperLimitTorqueForce=off  RyLowerLimitSpecify=on  RyLowerLimitBound=y_limits(1)  RyLowerLimitBoundUnits=deg  RyLowerLimitStiffness=1e4  RyLowerLimitStiffnessUnits=N*m/deg  RyLowerLimitDamping=10  RyLowerLimitDampingUnits=N*m/(deg/s)  RyLowerLimitTransitionRegionWidth=0.1  RyLowerLimitTransitionRegionWidthUnits=deg  RyUpperLimitSpecify=on  RyUpperLimitBound=y_limits(2)  RyUpperLimitBoundUnits=deg  RyUpperLimitStiffness=1e4  RyUpperLimitStiffnessUnits=N*m/deg  RyUpperLimitDamping=10  RyUpperLimitDampingUnits=N*m/(deg/s)  RyUpperLimitTransitionRegionWidth=0.1  RyUpperLimitTransitionRegionWidthUnits=deg  RyPositionTargetSpecify=on  RyPositionTargetPriority=High  RyPositionTargetValue=y_initial_position  RyPositionTargetValueUnits=deg  RyVelocityTargetSpecify=off  RyVelocityTargetPriority=High  RyVelocityTargetValue=0  RyVelocityTargetValueUnits=deg/s
  Viz Sphere : sm_lib/Body Elements/Spherical Solid  GraphicAmbientColor=[0.15 0.15 0.15 1.0]  BasedOnType=Mass  CenterOfMass=[0 0 0]  CenterOfMassUnits=m  GraphicDiffuseColor=color  Density=1000  DensityUnits=kg/m^3  DoExposeReferenceFrame=on  GraphicEmissiveColor=[0.0 0.0 0.0 1.0]  ExportEntireGeometry=off  SerializedExposedGeometries=<ExposedGeometries/>  SerializedFrames=<Frames/>  MarkerShape=Sphere  MarkerSize=10  GraphicType=FromGeometry  InertiaType=CalculateFromGeometry  Mass=0  MassUnits=kg  MomentsOfInertia=[1 1 1]  MomentsOfInertiaUnits=kg*m^2  GraphicOpacity=opacity  ProductsOfInertia=[0 0 0]  ProductsOfInertiaUnits=kg*m^2  GraphicShininess=75  GraphicSpecularColor=[0.5 0.5 0.5 1.0]  SphereRadius=radius  SphereRadiusUnits=m  GraphicVisPropType=SimpleVisualProperties
  F : PMIOPort  Side=Right
  B : PMIOPort  Port=2  Side=Left
  connections:
  Universal Joint/RConn1 -- F/RConn1
  B/RConn1 -- Universal Joint/LConn1 -- Viz Sphere/RConn1
